simulink model "Manoel_02"  (R2018a)
settings: Solver=VariableStepAuto  StartTime=0.0  StopTime=25  RelTol=1e-3
values from neighbouring files (symbols this model uses):
  atraso = stt    [manoel_outubro2.m]    (also in naao_roda.m = infor.SettlingTime; pre6_teste.m = infor.SettlingTime; pre_lab3.m = infor.SettlingTime; pre_lab3_lab.m = infor.SettlingTime)
  b0 = 18    [naao_roda.m]    (also in pre6_teste.m; pre_lab3.m; pre_lab3_2.m; pre_lab3_lab.m)
  ganho = 0.01027*infor.SettlingMax    [manoel_outubro2.m]    (also in naao_roda.m; pre6_teste.m; pre_lab3.m; pre_lab3_lab.m)
  R0 = round(r0,1)    [naao_roda.m]    (also in pre6_teste.m; pre_lab3.m; pre_lab3_lab.m; pre_lab4.m)
  T0 = round(t0,3)    [naao_roda.m]    (also in pre6_teste.m = 0.063; pre_lab3.m; pre_lab3_2.m = 0.0640576; pre_lab3_lab.m)
settings Model: Creator=joaovitor  LastModifiedBy=joaovitor

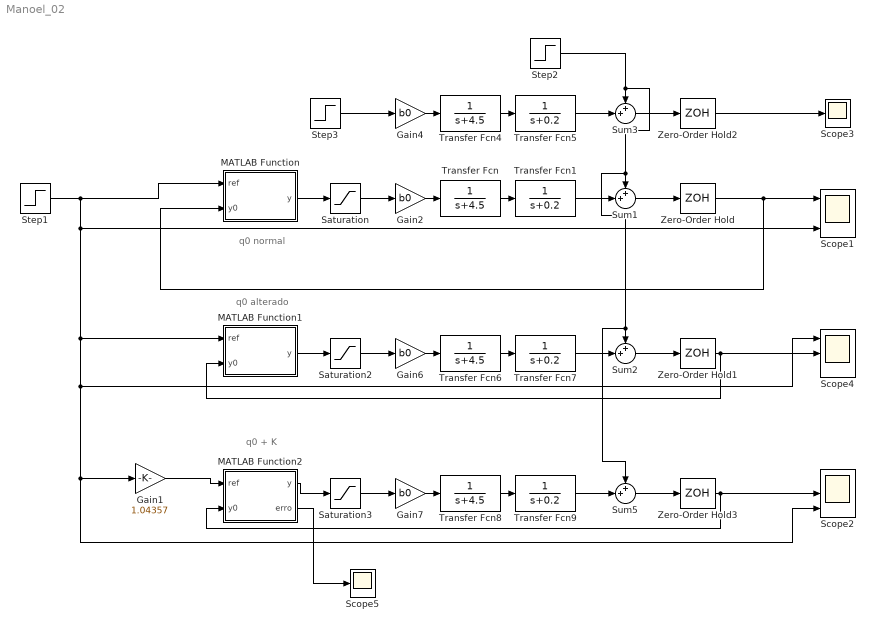
== system Manoel_02 ==
  note: q0 + K
  note: q0 alterado
  note: q0 normal
  Gain1 : Gain  Gain=1.04357
  Gain{2,4,6..7} (4 alike) : Gain  Gain=b0
  MATLAB Function : MATLAB Function  TreatAsAtomicUnit=on
  MATLAB Function1 : MATLAB Function  TreatAsAtomicUnit=on
  MATLAB Function2 : MATLAB Function  TreatAsAtomicUnit=on
  Saturation : Saturate  UpperLimit=10  LowerLimit=-10
  Saturation2 : Saturate  UpperLimit=10  LowerLimit=-10
  Saturation3 : Saturate  UpperLimit=10  LowerLimit=-10
  Scope1 : Scope  NumInputPorts=3
  Scope2 : Scope  NumInputPorts=3
  Scope3 : Scope
  Scope4 : Scope  NumInputPorts=3
  Scope5 : Scope
  Step1 : Step  Time=0  After=R0  SampleTime=0
  Step2 : Step  Time=3*atraso  After=10*ganho  SampleTime=0
  Step3 : Step  After=1.2  SampleTime=0
  Sum{1..3,5} (4 alike) : Sum  Inputs=++|
  Transfer Fcn{,4,6,8} (4 alike) : TransferFcn  Denominator=[1 4.5]
  Transfer Fcn{1,5,7,9} (4 alike) : TransferFcn  Denominator=[1 0.2]
  Zero-Order Hold{,1..3} (4 alike) : ZeroOrderHold  SampleTime=T0
  wires:
  Transfer Fcn/1 -> Transfer Fcn1/1
  Gain2/1 -> Transfer Fcn/1
  Zero-Order Hold/1 -> Scope1/1, MATLAB Function/2(y0)
  Sum1/1 -> Zero-Order Hold/1
  Transfer Fcn1/1 -> Sum1/2
  MATLAB Function/1(y) -> Saturation/1
  Saturation/1 -> Gain2/1
  Step1/1 -> MATLAB Function/1(ref), Scope1/3, Scope2/3, Gain1/1, Scope4/1, MATLAB Function1/1(ref)
  Step3/1 -> Gain4/1
  Gain4/1 -> Transfer Fcn4/1
  Transfer Fcn4/1 -> Transfer Fcn5/1
  Zero-Order Hold2/1 -> Scope3/1
  Sum3/1 -> Zero-Order Hold2/1
  Transfer Fcn5/1 -> Sum3/2
  Step2/1 -> Sum5/1, Sum2/1, Sum1/1, Sum3/1
  MATLAB Function2/1(y) -> Saturation3/1
  Saturation3/1 -> Gain7/1
  Gain7/1 -> Transfer Fcn8/1
  Transfer Fcn8/1 -> Transfer Fcn9/1
  MATLAB Function1/1(y) -> Saturation2/1
  Saturation2/1 -> Gain6/1
  Gain6/1 -> Transfer Fcn6/1
  Transfer Fcn6/1 -> Transfer Fcn7/1
  Transfer Fcn9/1 -> Sum5/2
  Transfer Fcn7/1 -> Sum2/2
  Sum5/1 -> Zero-Order Hold3/1
  Zero-Order Hold3/1 -> MATLAB Function2/2(y0), Scope2/2
  Sum2/1 -> Zero-Order Hold1/1
  Zero-Order Hold1/1 -> MATLAB Function1/2(y0), Scope4/2
  Gain1/1 -> MATLAB Function2/1(ref)
  MATLAB Function2/2(erro) -> Scope5/1

== matlab function Manoel_02/MATLAB Function1 ==
  data: ref input; y output; y0 input
function y = fcn(ref, y0)

ucontrole=(ref-y0)*1.14

y = ucontrole;


% O valor novo de q0 que reduz o erro pela metade é 1.14

% Eu mudei o tempo da perturbação para melhorar a visualização 

% Com o K igual a 1.086 a curva chega a 0.001 da ref

% Estou enviando com o K da letra d. O q0 de b foi comentado acima

== matlab function Manoel_02/MATLAB Function ==
  data: ref input; y output; y0 input
function y = fcn(ref, y0)

ucontrole=(ref-y0)*0.577

y = ucontrole;


% O valor novo de q0 que reduz o erro pela metade é 1.14

% Eu mudei o tempo da perturbação para melhorar a visualização 

% Com o K igual a 1.086 a curva chega a 0.001 da ref

% Estou enviando com o K da letra d. O q0 de b foi comentado acima

== matlab function Manoel_02/MATLAB Function2 ==
  data: ref input; y output; y0 input; erro output; R0 parameter
function [y,erro] = fcn(ref, y0, R0)

ucontrole=(ref-y0)*1.14

erro=(ref/R0)-y0

y = ucontrole;


% O valor novo de q0 que reduz o erro pela metade é 1.14

% Eu mudei o tempo da perturbação para melhorar a visualização 

% Com o K igual a 1.086 a curva chega a 0.001 da ref

% Estou enviando com o K da letra d. O q0 de b foi comentado acima
